simulink model "master"  (R2025a)
settings: Solver=VariableStepAuto  StartTime=0.0  StopTime=inf  RelTol=1e-3
values from neighbouring files (symbols this model uses):
  Boom_Cmd_LUT = joints(1).lut_y    [LUT.m]
  Boom_Vel_LUT = joints(1).lut_x    [LUT.m]
  Stick_Cmd_LUT = joints(2).lut_y    [LUT.m]
  Stick_Vel_LUT = joints(2).lut_x    [LUT.m]
undefined symbols (not defined in the file or in its folder): canChannel
libraries: canlib x10, canmsglib x8, simulink_extras x6, simulink x6, eeGeneralControl x5, slpidlib x5, aerolibanimutils x1, sl3dlib x1
(part 2 of 2)

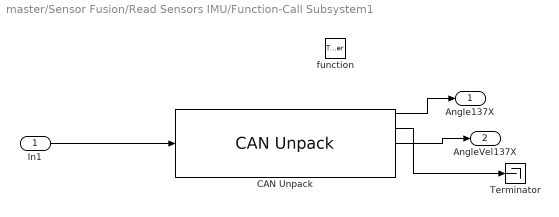
== system master/Sensor Fusion/Read Sensors IMU/Function-Call Subsystem1 ==
  In1 : Inport
  function : TriggerPort  TriggerType=function-call  VariantControl=(inherit)
  CAN Unpack : canmsglib/CAN Unpack  CANdbFile=.\dbc_files\ec20_kth.dbc  MsgList=IMU_XAxis_137  MsgName=IMU_XAxis_137  MsgIDType=Extended (29-bit identifier)  MsgIdentifier=251592841  MsgLength=8  SignalInfo={ 'AngleXAxis_137', '0', '16', 'LE', 'unsigned', 'Standard', '0', '0.007813', '0', '0', '512.025'; 'AngularAccelerationXAxis_137', '32', '16', 'LE', 'unsigned', 'Standard', '0', '0.03125', '-1000', '-1000', '1047.9688'; 'AngularVelocityXAxis_137', '16', '16', 'LE', 'unsigned', 'Standard', '0', '0.007813', '-250', '-250', '262.025'; 'CRC_Xaxis_137', '56', '8', 'LE', 'unsigned', 'Standard', '0', '1', '0', '0', '255'; 'Counter_Xaxis_137', '48', '8', 'LE', 'unsigned', 'Standard', '0', '1', '0', '0', '255' }  IDPort=off  TimestampPort=off  ErrorPort=off  RemotePort=off  LengthPort=off  StatusPort=off  ApplyMinMax=off
      settings: LibrarySourceBlock=canlib/CAN Unpack  DataFormat=CANdb specified signals
  Terminator : Terminator
  Angle137X : Outport
  AngleVel137X : Outport  Port=2
  wires:
  CAN Unpack/2 -> Terminator/1
  In1/1 -> CAN Unpack/1
  CAN Unpack/1 -> Angle137X/1
  CAN Unpack/3 -> AngleVel137X/1

== system master/Sensor Fusion/Read Sensors IMU/Function-Call Subsystem2 ==
  In1 : Inport
  function : TriggerPort  TriggerType=function-call  VariantControl=(inherit)
  CAN Unpack : canmsglib/CAN Unpack  CANdbFile=.\dbc_files\ec20_kth.dbc  MsgList=IMU_XAxis_138  MsgName=IMU_XAxis_138  MsgIDType=Extended (29-bit identifier)  MsgIdentifier=251592842  MsgLength=8  SignalInfo={ 'AngleXAxis_138', '0', '16', 'LE', 'unsigned', 'Standard', '0', '0.007813', '0', '0', '512.025'; 'AngularAccelerationXAxis_138', '32', '16', 'LE', 'unsigned', 'Standard', '0', '0.03125', '-1000', '-1000', '1047.9688'; 'AngularVelocityXAxis_138', '16', '16', 'LE', 'unsigned', 'Standard', '0', '0.007813', '-250', '-250', '262.025'; 'CRC_Xaxis_138', '56', '8', 'LE', 'unsigned', 'Standard', '0', '1', '0', '0', '255'; 'Counter_Xaxis_138', '48', '8', 'LE', 'unsigned', 'Standard', '0', '1', '0', '0', '255' }  IDPort=off  TimestampPort=off  ErrorPort=off  RemotePort=off  LengthPort=off  StatusPort=off  ApplyMinMax=off
      settings: LibrarySourceBlock=canlib/CAN Unpack  DataFormat=CANdb specified signals
  Terminator : Terminator
  Angle138X : Outport
  AngleVel138X : Outport  Port=2
  wires:
  CAN Unpack/2 -> Terminator/1
  CAN Unpack/1 -> Angle138X/1
  In1/1 -> CAN Unpack/1
  CAN Unpack/3 -> AngleVel138X/1

== system master/Sensor Fusion/Read Sensors IMU/Function-Call Subsystem3 ==
  In1 : Inport
  function : TriggerPort  TriggerType=function-call  VariantControl=(inherit)
  CAN Unpack : canmsglib/CAN Unpack  CANdbFile=.\dbc_files\ec20_kth.dbc  MsgList=IMU_XAxis_139  MsgName=IMU_XAxis_139  MsgIDType=Extended (29-bit identifier)  MsgIdentifier=251592843  MsgLength=8  SignalInfo={ 'AngleXAxis_139', '0', '16', 'LE', 'unsigned', 'Standard', '0', '0.007813', '0', '0', '512.025'; 'AngularAccelerationXAxis_139', '32', '16', 'LE', 'unsigned', 'Standard', '0', '0.03125', '-1000', '-1000', '1047.9688'; 'AngularVelocityXAxis_139', '16', '16', 'LE', 'unsigned', 'Standard', '0', '0.007813', '-250', '-250', '262.025'; 'CRC_Xaxis_139', '56', '8', 'LE', 'unsigned', 'Standard', '0', '1', '0', '0', '255'; 'Counter_Xaxis_139', '48', '8', 'LE', 'unsigned', 'Standard', '0', '1', '0', '0', '255' }  IDPort=off  TimestampPort=off  ErrorPort=off  RemotePort=off  LengthPort=off  StatusPort=off  ApplyMinMax=off
      settings: LibrarySourceBlock=canlib/CAN Unpack  DataFormat=CANdb specified signals
  Terminator : Terminator
  Angle139X : Outport
  AngleVel139X : Outport  Port=2
  wires:
  CAN Unpack/3 -> AngleVel139X/1
  In1/1 -> CAN Unpack/1
  CAN Unpack/1 -> Angle139X/1
  CAN Unpack/2 -> Terminator/1

== matlab function master/Sensor Fusion/MATLAB Function1 ==
  data: EncoderPos20X input; angle_20 output; EncoderVel20X input; joint2_pos input; joint2_vel input; velocity_20 output
function [angle_20, velocity_20]= kalman_block(EncoderPos20X, EncoderVel20X, joint2_pos, joint2_vel)
    persistent kf_20
    if isempty(kf_20)
        kf_20 = KalmanFilter(0.01);
    end
    
    kf_20.predict();
    kf_20.update(EncoderPos20X, EncoderVel20X, joint2_pos, joint2_vel);
    
    angle_20 = kf_20.x(1);
    velocity_20 = kf_20.x(2);

end

== matlab function master/Sensor Fusion/MATLAB Function ==
  data: EncoderPos33X input; angle_33 output; EncoderVel33X input; joint1_pos input; joint1_vel input; velocity_33 output
function [angle_33, velocity_33]= kalman_block(EncoderPos33X, EncoderVel33X, joint1_pos, joint1_vel)
    persistent kf_33
    if isempty(kf_33)
        kf_33 = KalmanFilter(0.01);
    end

    kf_33.predict();
    kf_33.update(EncoderPos33X, EncoderVel33X, joint1_pos, joint1_vel);
    
    angle_33 = kf_33.x(1);
    velocity_33 = kf_33.x(2);

end

== matlab function master/Sensor Fusion/MATLAB Function2 ==
  data: EncoderPos01X input; angle_01 output; EncoderVel01X input; joint3_pos input; joint3_vel input; velocity_01 output
function [angle_01, velocity_01]= kalman_block(EncoderPos01X, EncoderVel01X, joint3_pos, joint3_vel)
    persistent kf_01
    if isempty(kf_01)
        kf_01 = KalmanFilter(0.01);
    end
    
    kf_01.predict();
    kf_01.update(EncoderPos01X, EncoderVel01X, joint3_pos, joint3_vel);
    
    angle_01 = kf_01.x(1);
    velocity_01 = kf_01.x(2);

end

== matlab function master/controller/inverse_kinematics ==
  data: vx_ref input; thetadot_ref output; vy_ref input; theta1 input; theta2 input
function thetadot_ref = fcn(vx_ref, vy_ref, theta1, theta2)
% Safe version for Simulink — works even when inputs become vectors

vx_ref = vx_ref(1);


% Link lengths [m]
L1 = 1903.392e-3;
L2 = 1351.485e-3;

max_joint_vel1 = 0.1;  
max_joint_vel2 = 0.1;

% --- Jacobian ---
J11 = -L1 * sin(theta1) - L2 * sin(theta1 + theta2);
J12 = -L2 * sin(theta1 + theta2);
J21 =  L1 * cos(theta1) + L2 * cos(theta1 + theta2);
J22 =  L2 * cos(theta1 + theta2);

J = [J11 J12; 
     J21 J22];

% --- desired Cartesian velocity vector (2×1) ---
xydot_ref = [vx_ref; vy_ref];



% --- compute damped least squares inverse (2x2 case) ---
lambda = 0.05;   % damping, tune (0.01..0.2) as needed
JJt = J * J';
inv_term = inv(JJt + lambda^2 * eye(2));
J_dls = J' * inv_term;

thetadot = J_dls * xydot_ref;

% --- clip to joint velocity limits ---
thetadot1 = max(min(thetadot(1), max_joint_vel1), -max_joint_vel1);
thetadot2 = max(min(thetadot(2), max_joint_vel2), -max_joint_vel2);

% --- output vector (2×1) ---
thetadot_ref = [thetadot1; thetadot2];
end

== matlab function master/calculate_position ==
  data: x output; theta1 input; y output; theta2 input
function [x,y]= fcn(theta1, theta2)

L1 = 1903.392e-3;
L2 = 1351.485e-3;

x = L1*cos(theta1) + L2*cos(theta1 + theta2);
x1 = L1*cos(theta1) + L2*cos(2*pi - theta1 - theta2);


y = L1*sin(theta1) + L2*sin(theta1 + theta2);
y1 = L1*sin(theta1) - L2*sin(2*pi - theta1 - theta2);
y2 = L1*sin(theta1) + L2*sin(2*pi - theta1 - theta2);

== matlab function master/calculate_velocity ==
  data: theta1dot input; xdot output; theta2dot input; ydot output; theta1 input; theta2 input
function [xdot, ydot] = fcn(theta1dot, theta2dot, theta1, theta2)

% Link lengths [m]
L1 = 1903.392e-3;
L2 = 1351.485e-3;


% --- Jacobian ---
J11 = -L1 * sin(theta1) - L2 * sin(theta1 + theta2);
J12 = -L2 * sin(theta1 + theta2);
J21 =  L1 * cos(theta1) + L2 * cos(theta1 + theta2);
J22 =  L2 * cos(theta1 + theta2);

J = [J11 J12; 
     J21 J22];
xydot = J*[theta1dot; theta2dot];

xdot = xydot(1);
ydot = xydot(2);
